simulink model "RBNN_Nonlinear_system_3layer_system2_multimodal"  (R2019a)
settings: Solver=VariableStepAuto  StartTime=0.0  StopTime=inf  FixedStep=0.001  RelTol=1e-3
libraries: simulink x1
settings Model: Creator=vardhah  LastModifiedBy=vardhah
settings DataIOCC: ReturnWorkspaceOutputs=off
settings DebuggingCC: UnderSpecifiedDimensionMsg=warning  ArithmeticOperatorsInVariantConditions=warning

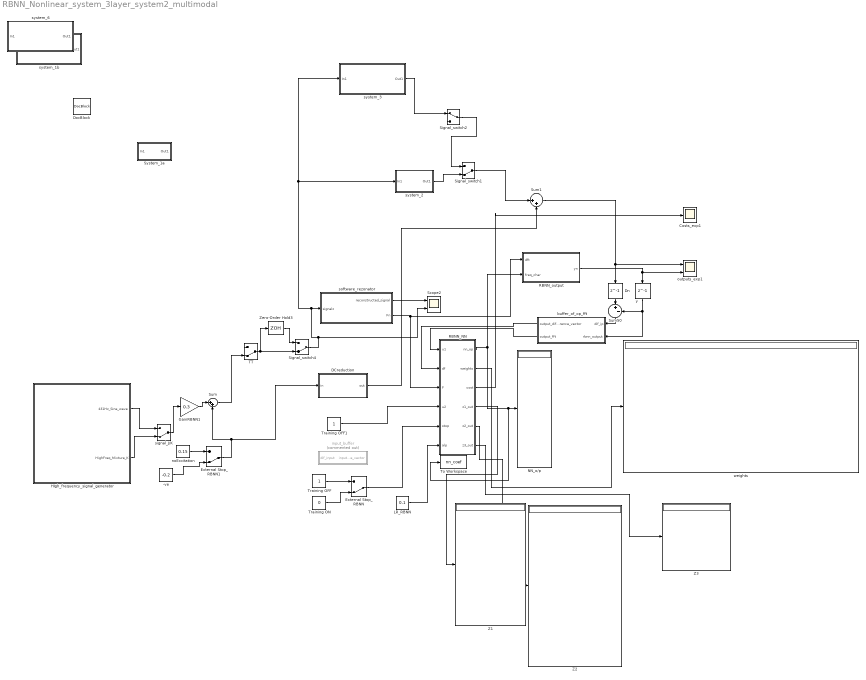
== system RBNN_Nonlinear_system_3layer_system2_multimodal ==
  -ve : Constant  Value=-0.2
  Costs_exp1 : Scope
  DCreduction : MATLAB Function  TreatAsAtomicUnit=on
  Dn : Delay  DelayLength=1  InitialCondition=0
  DocBlock : simulink/Model-Wide Utilities/DocBlock  DocumentType=Text
      content=|
      | system 3: gain = 0.5
      |
      | system 6: gain = 0.4
      |
      | system 1b : gain= 0.2
      |
      | Training signal 373+498 rads/ s ( amplitude 0.5)
      |
      | Testing signal 1098+1431 rad/s (amplitude 0.5)
  External Stop_RBNN : ManualSwitch  CurrentSetting=0
  External Stop_RBNN1 : ManualSwitch  CurrentSetting=0
  GainRBNN1 : Gain  Gain=0.3
  HIgh_frequency_signal_generator : Subsystem
  LR_RBNN : Constant  Value=0.1
  NN_o/p : Display
  RBNN_NN : MATLAB Function  TreatAsAtomicUnit=on
  RBNN_output : MATLAB Function  TreatAsAtomicUnit=on
  Scope2 : Scope  NumInputPorts=2
  Signal_switch1 : ManualSwitch  CurrentSetting=0
  Signal_switch2 : ManualSwitch
  Signal_switch4 : ManualSwitch  CurrentSetting=0
  Sum : Sum  Inputs=|++
  Sum1 : Sum  Inputs=|++
  Sum50 : Sum  Inputs=|+-
  System_1a : Subsystem
  TT : ManualSwitch  CurrentSetting=0
  To Workspace : ToWorkspace  VariableName=nn_coef  SaveFormat=Timeseries  SampleTime=-1
  Training OFF : Constant
  Training OFF1 : Constant
  Training ON : Constant  Value=0
  Z1 : Display
  Z2 : Display
  Z3 : Display
  Zero-Order Hold3 : ZeroOrderHold  SampleTime=0.0001
  buffer_of_op_fft : MATLAB Function  TreatAsAtomicUnit=on
  input_buffer : MATLAB Function  Commented=on  TreatAsAtomicUnit=on
  noExcitation : Constant  Value=0.15
  outputs_exp1 : Scope  NumInputPorts=2
  signal_J/K : ManualSwitch  CurrentSetting=0
  software_rezonator : MATLAB Function  TreatAsAtomicUnit=on
  system_1b : Subsystem
  system_2 : Subsystem
  system_3 : Subsystem
  system_6 : Subsystem
  weights : Display
  y : Delay  DelayLength=1  InitialCondition=0
  wires:
  software_rezonator/1(reconstructed_signal) -> Scope2/1
  software_rezonator/2(Fn) -> RBNN_NN/3(F), RBNN_output/1(dft)
  Dn/1 -> Sum50/1
  y/1 -> buffer_of_op_fft/2(rbnn_output), Sum50/2
  RBNN_NN/1(nn_op) -> To Workspace/1, NN_o/p/1, RBNN_output/2(freq_char)
  External Stop_RBNN/1 -> RBNN_NN/5(stop)
  Training OFF/1 -> External Stop_RBNN/1
  Training ON/1 -> External Stop_RBNN/2
  RBNN_NN/3(cost) -> Costs_exp1/1
  RBNN_NN/2(weights) -> weights/1
  RBNN_NN/4(z1_out) -> Z1/1
  Sum50/1 -> buffer_of_op_fft/1(dif_ip)
  buffer_of_op_fft/1(output_difference_vector) -> RBNN_NN/2(df)
  buffer_of_op_fft/2(output_fft) -> RBNN_NN/1(u1)
  TT/1 -> Zero-Order Hold3/1, Signal_switch4/2
  LR_RBNN/1 -> RBNN_NN/6(alp)
  HIgh_frequency_signal_generator/1(431Hz_Sine_wave) -> signal_J/K/1
  HIgh_frequency_signal_generator/2(HighFreq_Mixture_K) -> signal_J/K/2
  signal_J/K/1 -> GainRBNN1/1
  Zero-Order Hold3/1 -> Signal_switch4/1
  Signal_switch4/1 -> Scope2/2, system_2/1(In1), system_3/1(In1), software_rezonator/1(signalz)
  Signal_switch1/1 -> Sum1/1
  Sum1/1 -> outputs_exp1/1, Dn/1
  Training OFF1/1 -> RBNN_NN/4(u2)
  RBNN_NN/5(z2_out) -> Z2/1
  RBNN_NN/6(z3_out) -> Z3/1
  RBNN_output/1(yn) -> outputs_exp1/2, y/1
  system_3/1(Out1) -> Signal_switch2/1
  Signal_switch2/1 -> Signal_switch1/1
  system_2/1(Out1) -> Signal_switch1/2
  GainRBNN1/1 -> Sum/1
  Sum/1 -> TT/2
  External Stop_RBNN1/1 -> Sum/2, DCreduction/1(in)
  noExcitation/1 -> External Stop_RBNN1/1
  -ve/1 -> External Stop_RBNN1/2
  DCreduction/1(out) -> Sum1/2

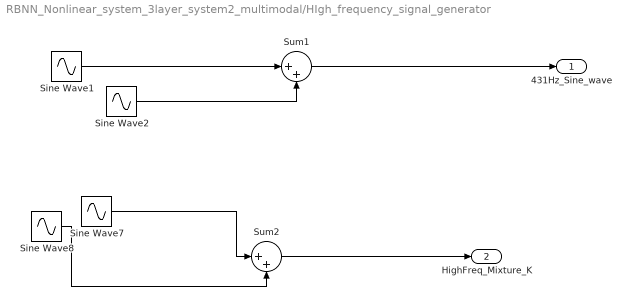
== system RBNN_Nonlinear_system_3layer_system2_multimodal/HIgh_frequency_signal_generator ==
  Sine Wave1 : Sin  Amplitude=0.5  Frequency=1431  SampleTime=0
  Sine Wave2 : Sin  Amplitude=0.5  Frequency=1098  SampleTime=0
  Sine Wave7 : Sin  Amplitude=0.4  Frequency=537  SampleTime=0
  Sine Wave8 : Sin  Amplitude=0.4  Frequency=373  SampleTime=0
  Sum1 : Sum  Inputs=|++
  Sum2 : Sum  Inputs=|++
  431Hz_Sine_wave : Outport
  HighFreq_Mixture_K : Outport  Port=2
  wires:
  Sine Wave7/1 -> Sum2/1
  Sine Wave8/1 -> Sum2/2
  Sum2/1 -> HighFreq_Mixture_K/1
  Sine Wave1/1 -> Sum1/1
  Sine Wave2/1 -> Sum1/2
  Sum1/1 -> 431Hz_Sine_wave/1

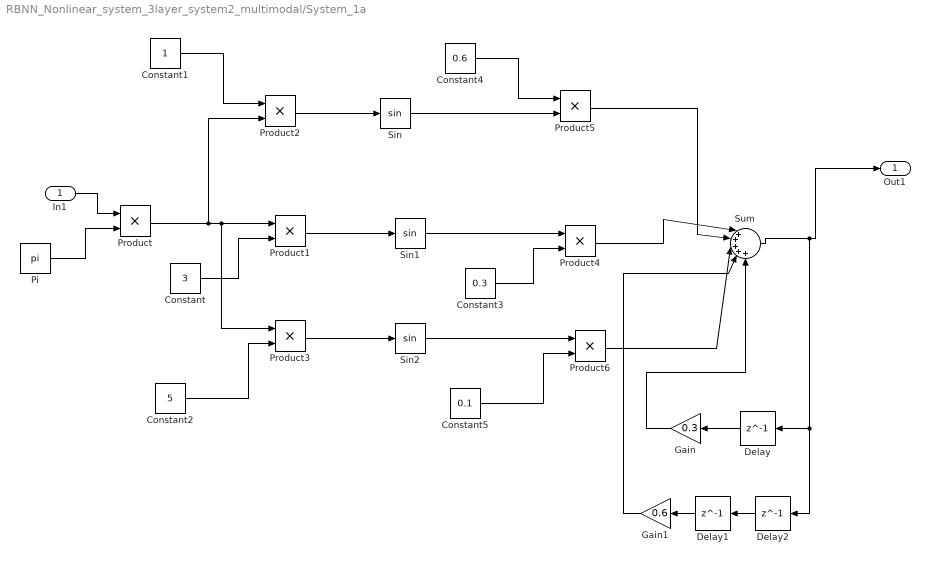
== system RBNN_Nonlinear_system_3layer_system2_multimodal/System_1a ==
  In1 : Inport
  Constant : Constant  Value=3
  Constant1 : Constant
  Constant2 : Constant  Value=5
  Constant3 : Constant  Value=0.3
  Constant4 : Constant  Value=0.6
  Constant5 : Constant  Value=0.1
  Delay : Delay  DelayLength=1  InitialCondition=0
  Delay1 : Delay  DelayLength=1  InitialCondition=0
  Delay2 : Delay  DelayLength=1  InitialCondition=0
  Gain : Gain  Gain=0.3
  Gain1 : Gain  Gain=0.6
  Pi : Constant  Value=pi  OutDataTypeStr=Inherit: Inherit via back propagation
  Product{,1..6} (7 alike) : Product
  Sin : Trigonometry
  Sin1 : Trigonometry
  Sin2 : Trigonometry
  Sum : Sum  Inputs=|+++++
  Out1 : Outport
  wires:
  Pi/1 -> Product/2
  In1/1 -> Product/1
  Constant1/1 -> Product2/1
  Product/1 -> Product2/2, Product3/1, Product1/1
  Constant/1 -> Product1/2
  Constant2/1 -> Product3/2
  Product2/1 -> Sin/1
  Product3/1 -> Sin2/1
  Product1/1 -> Sin1/1
  Product5/1 -> Sum/2
  Constant4/1 -> Product5/1
  Product6/1 -> Sum/3
  Constant5/1 -> Product6/2
  Constant3/1 -> Product4/2
  Product4/1 -> Sum/1
  Sin1/1 -> Product4/1
  Sin/1 -> Product5/2
  Sin2/1 -> Product6/1
  Sum/1 -> Delay/1, Delay2/1, Out1/1
  Delay2/1 -> Delay1/1
  Delay/1 -> Gain/1
  Delay1/1 -> Gain1/1
  Gain/1 -> Sum/5
  Gain1/1 -> Sum/4

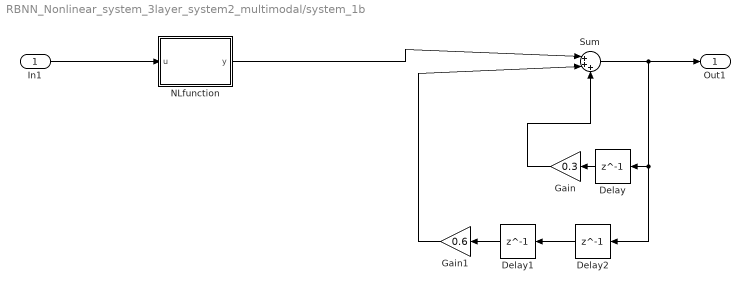
== system RBNN_Nonlinear_system_3layer_system2_multimodal/system_1b ==
  In1 : Inport
  Delay : Delay  DelayLength=1  InitialCondition=0
  Delay1 : Delay  DelayLength=1  InitialCondition=0
  Delay2 : Delay  DelayLength=1  InitialCondition=0
  Gain : Gain  Gain=0.3
  Gain1 : Gain  Gain=0.6
  NLfunction : MATLAB Function  TreatAsAtomicUnit=on
  Sum : Sum  Inputs=|+++
  Out1 : Outport
  wires:
  In1/1 -> NLfunction/1(u)
  Delay2/1 -> Delay1/1
  Sum/1 -> Delay2/1, Delay/1, Out1/1
  Delay/1 -> Gain/1
  Delay1/1 -> Gain1/1
  NLfunction/1(y) -> Sum/1
  Gain/1 -> Sum/3
  Gain1/1 -> Sum/2

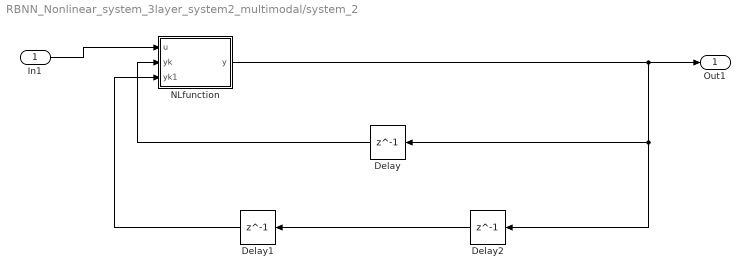
== system RBNN_Nonlinear_system_3layer_system2_multimodal/system_2 ==
  In1 : Inport
  Delay : Delay  DelayLength=1  InitialCondition=0
  Delay1 : Delay  DelayLength=1  InitialCondition=0
  Delay2 : Delay  DelayLength=1  InitialCondition=0
  NLfunction : MATLAB Function  TreatAsAtomicUnit=on
  Out1 : Outport
  wires:
  In1/1 -> NLfunction/1(u)
  Delay2/1 -> Delay1/1
  NLfunction/1(y) -> Out1/1, Delay2/1, Delay/1
  Delay/1 -> NLfunction/2(yk)
  Delay1/1 -> NLfunction/3(yk1)

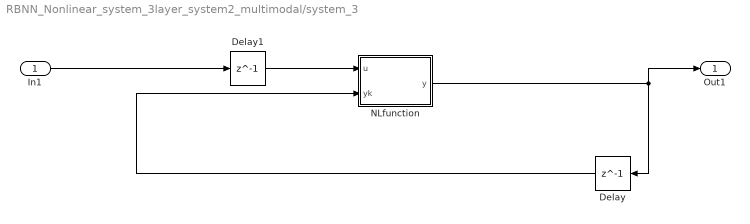
== system RBNN_Nonlinear_system_3layer_system2_multimodal/system_3 ==
  In1 : Inport
  Delay : Delay  DelayLength=1  InitialCondition=0
  Delay1 : Delay  DelayLength=1  InitialCondition=0
  NLfunction : MATLAB Function  TreatAsAtomicUnit=on
  Out1 : Outport
  wires:
  In1/1 -> Delay1/1
  NLfunction/1(y) -> Out1/1, Delay/1
  Delay/1 -> NLfunction/2(yk)
  Delay1/1 -> NLfunction/1(u)

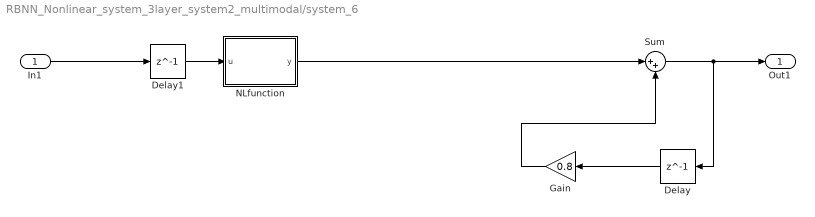
== system RBNN_Nonlinear_system_3layer_system2_multimodal/system_6 ==
  In1 : Inport
  Delay : Delay  DelayLength=1  InitialCondition=0
  Delay1 : Delay  DelayLength=1  InitialCondition=0
  Gain : Gain  Gain=0.8
  NLfunction : MATLAB Function  TreatAsAtomicUnit=on
  Sum : Sum  Inputs=|++
  Out1 : Outport
  wires:
  In1/1 -> Delay1/1
  Sum/1 -> Delay/1, Out1/1
  Delay/1 -> Gain/1
  NLfunction/1(y) -> Sum/1
  Gain/1 -> Sum/2
  Delay1/1 -> NLfunction/1(u)

== matlab function RBNN_Nonlinear_system_3layer_system2_multimodal/system_1b/NLfunction ==
  data: u input; y output
function y = fcn(u)

y = u^3+0.3*u^2-0.4*u;
end

== matlab function RBNN_Nonlinear_system_3layer_system2_multimodal/RBNN_NN ==
  settings: sampleTime=0.01
  data: u1 input; df input; F input; u2 input; nn_op output; weights output; cost output; z1_out output; stop input; alp input; z2_out output; z3_out output
function [nn_op,weights,cost,z1_out,z2_out,z3_out]  = NN(u1,df,F,u2,stop,alp)

persistent w1 w2 w3;
persistent vy;
persistent g1 g2 g3;
persistent itr;
persistent J;
persistent del_w1 del_w2 del_w3;
persistent mult1 mult2 mult3;
persistent memory_alloc_flag;
persistent n;

%%
%%%%%%----------------------------------------------------------------------------%%%%%
%Hyper-parameter & other tunable part of code

M=1;   %declare batch size of training (It will also be equal to number of input in our case as we are using DFT)
E=1;    % size of external associative input

%layer declaration
layer_1=32;
layer_2=32;
layer_3=8;       % Output layer must match with number of rezonators declared in rezonator function

%learning rate. Currently reading from input pin 
alpha = alp;

%others
input_layer =M+E;       %layer_0
output_layer=layer_3;

% weight Intialisation 
if isempty(w1)
       w1=randn(input_layer,layer_1)*0.1;
end
if isempty(w2)
       w2=randn(layer_1,layer_2)*0.1;
end
if isempty(w3)
       w3=randn(layer_2,layer_3)*0.1;
end

%%%%%---------------------------------------------------------------------------------%%%%%

%%

%synchronising clock
if isempty(n)
        n = 0; end
n=n+1;

%%
%Allocation of variables that will be used during runtime( one time execution code) 
if isempty(memory_alloc_flag)
        memory_alloc_flag = 0; 
end
if isempty(mult1)
       mult1=zeros(layer_1,layer_1*input_layer); 
end
if isempty(mult2)
       mult2=zeros(layer_2,layer_1*layer_2); 
end
if isempty(mult3)
       mult3=zeros(layer_3,layer_2*layer_3); 
end
if isempty(vy)
       vy=zeros(input_layer,M); 
end

if memory_alloc_flag==0
 %write memory allocation for looped code here.It runs once and store it in memory.  
 mult1=[];
 mult2=[];
 mult3=[];
  for iteration =1:layer_1
   mult1=[mult1;[zeros(1,(iteration-1)*input_layer) ones(1,input_layer) zeros(1,(layer_1-iteration)*input_layer)]];
  end
  for iterate=1:layer_2
   mult2=[mult2;[zeros(1,(iterate-1)*layer_1) ones(1,layer_1) zeros(1,(layer_2-iterate)*layer_1)]];
  end
  for iterate=1:layer_3
   mult3=[mult3;[zeros(1,(iterate-1)*layer_2) ones(1,layer_2) zeros(1,(layer_3-iterate)*layer_2)]];
  end
 
 for k= 1:input_layer
    for j = 1:M 
        if k<=(M/2)+1 && k>=1
            vy(k,j)=(1/M)*cos(pi*(M-j)*(k-1)/(M/2));
        elseif k<=M && k>=(M/2)+1
            vy(k,j)=-(1/M)*sin(pi*(M-j)*(k-1)/(M/2));
        elseif k>M
            vy(k,j)=0;     
        end
    end
 end
 memory_alloc_flag=1; 
end

%%
%============All other Initiaisation =========================>

%Initialisation of delta of weight storage
if isempty(del_w1)
    del_w1=zeros(1,input_layer*layer_1);
end
if isempty(del_w2)
    del_w2=zeros(1,layer_2*layer_1);
end
if isempty(del_w3)
    del_w3=zeros(1,layer_2*layer_3);
end

%Intialising iteration number & cost value. 
if isempty(itr)
    itr=0;
end
if isempty(J)
    J=0;
end


%gradient initialisation(in matrix form)
if isempty(g1)
    g1= zeros(M,input_layer*layer_1);   
end
if isempty(g2)
    g2= zeros(M,layer_1*layer_2);   
end
if isempty(g3)
    g3= zeros(M,layer_3*layer_2);   
end

%%
%Input vector creation code block
x_in = [real(u1(1:(size(u1,2)/2)+1)) imag(u1(1:(size(u1,2)/2)-1))];
v=transpose([x_in transpose(u2)]);

%%
%RBNN core vectorised algorithm implementation 

%--------------->forward propogation ------------>

z1=w1'*v ;
a1=(1./(1+exp(-z1)));
an1=(a1-0.5);
z2=w2'*an1 ;
a2=(1./(1+exp(-z2)));
an2=(a2-0.5);
z3=w3'*an2 ;
a3=(1./(1+exp(-z3)));
an3=(a3-0.5)*2;

%-------------> Backward Propogation -------->

%calculation of Nv:
da3_z3=a3.*(1-a3);
dn_a2=w3'.*repmat(da3_z3,1,layer_2);
da2_z2=a2.*(1-a2);
dn_z2= dn_a2.* repmat(transpose(da2_z2),output_layer,1);
dn_a1=dn_z2*w2';
da1_z1=a1.*(1-a1); 
dn_z1=dn_a1.*repmat(transpose(da1_z1),output_layer,1);
dn_v=dn_z1*w1';   %"This is Nv" 

%calculation of aD, A & B 
aD=transpose(F)*dn_v*vy;
A=[aD;eye(M-1) zeros(M-1,1)];
B=[transpose(F) ; zeros(M-1,size(F,1))]; 

%calculation of Nw(diff of N(v,w) wrt each weights)
dIn_3= da3_z3*transpose(a2);
dn_w3=repmat(dIn_3,1,layer_3).* mult3;

dIn_2= da2_z2*transpose(a1);
da2_w2=repmat(dIn_2,1,layer_2).* mult2;
dn_w2=dn_a2*da2_w2;

dIn_1= da1_z1*transpose(v);
da1_w1= repmat(dIn_1,1,layer_1).*mult1;
dn_w1=dn_a1*da1_w1;

%gradient updation
g3=A*g3+B*dn_w3;
g2=A*g2+B*dn_w2;
g1=A*g1+B*dn_w1;

%Training & updation only once in a batch(batch size=M,n=Overall counter) 
if mod(n,M)==0 && stop==0
    del_w1 =alpha*df*1*g1/M ;
    del_w2 =alpha*df*1*g2/M ;
    del_w3 =alpha*df*1*g3/M ;
    del_w_reshaped1= reshape(del_w1,[input_layer,layer_1]);
    del_w_reshaped2= reshape(del_w2,[layer_1,layer_2]);
    del_w_reshaped3= reshape(del_w3,[layer_2,layer_3]);
    w1=w1+ del_w_reshaped1;
    w2=w2+ del_w_reshaped2;
    w3=w3+ del_w_reshaped3; 
    itr=itr+1;
    J= sum(df.^2,'all')/(2*M);
end

%For logging & visulisation purpose
cost=J;
weights=w1;
z1_out=z1;
z2_out=z2;
z3_out=z3;

%NN output assignment
nn_op=an3;


end

== matlab function RBNN_Nonlinear_system_3layer_system2_multimodal/buffer_of_op_fft ==
  data: output_difference_vector output size=[1,1]; output_fft output size=[1,1]; dif_ip input; rbnn_output input
function [output_difference_vector,output_fft] = difBuffer(dif_ip,rbnn_output)                      

 sz=1;                       % size of the dft 
 
 persistent a;
 persistent b;
 if isempty(b)
  b= zeros(1,sz);
 end
 if isempty(a)
  a= zeros(1,sz);
 end
 
 
  a= circshift(a,1);
  a(1)=dif_ip;
  b= circshift(b,1);
  b(1)=rbnn_output;

 output_difference_vector=a; 
 output_fft=1/sz*fft(b); 
end

== matlab function RBNN_Nonlinear_system_3layer_system2_multimodal/input_buffer ==
  data: input_difference_vector output size=[1,16]; dif_input input
function input_difference_vector  = difBuffer(dif_input)                      

 sz=16;                       % size of the dft 
 
 persistent a;
 if isempty(a)
  a= zeros(1,sz);
 end
 
 
  a= circshift(a,1);
  a(1)=dif_input;
 input_difference_vector=a; 
end

== matlab function RBNN_Nonlinear_system_3layer_system2_multimodal/system_6/NLfunction ==
  data: u input; y output
function y = fcn(u)

y = (u-0.8)*u*(u+0.5);
end

== matlab function RBNN_Nonlinear_system_3layer_system2_multimodal/system_3/NLfunction ==
  data: u input; y output; yk input
function y = fcn(u, yk)

y = (yk/(1+yk^2)) + u^3;
end

== matlab function RBNN_Nonlinear_system_3layer_system2_multimodal/software_rezonator ==
  data: signalz input; reconstructed_signal output size=1; Fn output size=8
function [reconstructed_signal,Fn]   = rezonator(signalz)

persistent numberofrezonator;
persistent g c bfr_rezo_sm aft_delay dft_out;
persistent out signal_dif;
persistent n;
persistent memory_alloc_flag;


%assign the number of rezonator here. For configuring it for higher order
%rezonator  we need to change (1) 'numberofrezonaotor' variable
if isempty(numberofrezonator)
        numberofrezonator = 8;   %here 16 parallel rezonators
end
N=8;
%Initialisation of memory allocations/variables ====> 
if isempty(memory_alloc_flag)
        memory_alloc_flag = 0; 
end
if isempty(g)
       g=zeros(numberofrezonator,numberofrezonator,'like',0i); 
end
if isempty(c)
       c=zeros(numberofrezonator,numberofrezonator,'like',0i); 
end
if memory_alloc_flag==0
 for i=0:numberofrezonator-1
  for j= 0:numberofrezonator-1
   g(i+1,j+1)=1/numberofrezonator*(exp(-1i*2*pi*i*j/numberofrezonator));
   c(i+1,j+1)=(exp(1i*2*pi*i*j/numberofrezonator));
  end 
 end
 memory_alloc_flag=1;
end


%Initialisation of variables  =====> 
if isempty(n)
        n = 0;   
end 
if isempty(out)
  out=0+0i;
end
if isempty(signal_dif)
  signal_dif=0+0i;
end
if isempty(bfr_rezo_sm)
  bfr_rezo_sm=repmat(0+0i,numberofrezonator,1);
end
if isempty(aft_delay)
  aft_delay=repmat(0+0i,numberofrezonator,1);
end
if isempty(dft_out)
  dft_out=repmat(0+0i,numberofrezonator,1);
end

%creating cycle of rotation for selection of correct column of g & c.
cycle=mod(n,numberofrezonator);

%resonator core -----------------------------> 
dft_out=c(:,cycle+1).*aft_delay;
out= sum(dft_out,1);
signal_dif=signalz-out;
bfr_rezo_sm=g(:,cycle+1).*signal_dif;

%counting the counter
n=n+1;

% output assignment ------------------>
reconstructed_signal=out;
dft=aft_delay; 
%N=size(dft,1);
a=1:1:N/2-1;
b=N/2+1:1:N-1;
dft_trans=transpose(dft);
Fn=transpose([real(dft_trans(1)) 2*(real(dft_trans(2:N/2)).*cos(2*pi*a*n/N)-imag(dft_trans(2:N/2)).*sin(2*pi*a*n/N)) -1^n*real(dft_trans(N/2+1)) -2*(imag(dft_trans(N/2+2:N)).*cos(2*pi*b*n/N)+real(dft_trans(N/2+2:N)).*sin(2*pi*b*n/N))]);
%--------output assignment over----------<

%final updation of buffer ------>>>>>>>>>>>>
aft_delay= aft_delay+bfr_rezo_sm; 
end

== matlab function RBNN_Nonlinear_system_3layer_system2_multimodal/RBNN_output ==
  data: dft input; yn output; freq_char input
function yn = fcn(dft,freq_char)
yn=transpose(freq_char)*dft;
end

== matlab function RBNN_Nonlinear_system_3layer_system2_multimodal/system_2/NLfunction ==
  data: u input; yk input; yk1 input; y output
function y = fcn(u,yk, yk1)

a = (yk*yk1*(yk+2.5))/(1+yk^2+yk1^2);
y = a+u;
end

== matlab function RBNN_Nonlinear_system_3layer_system2_multimodal/DCreduction ==
  data: out output; in input
function out  = difBuffer(in)                      

if in==-0.2
    out = 0;
else 
    out =-2.5;
end
